simulink model "otonom_sim_lane_changing"  (R2021b)
settings: Solver=VariableStepAuto  StartTime=0.0  StopTime=100  RelTol=1e-3
libraries: simulink x16, sim3dcameralib x8, eeGeneralControl x4, robotmobilelib x2, sim3dautolib x2, slpidlib x1, sim3dlib x1
settings Model: Creator=Asus  LastModifiedBy=cx

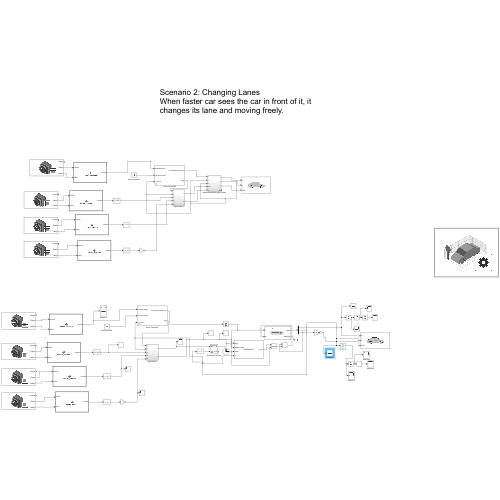
[thumbnail: Simulink's stored preview of the top-level diagram]
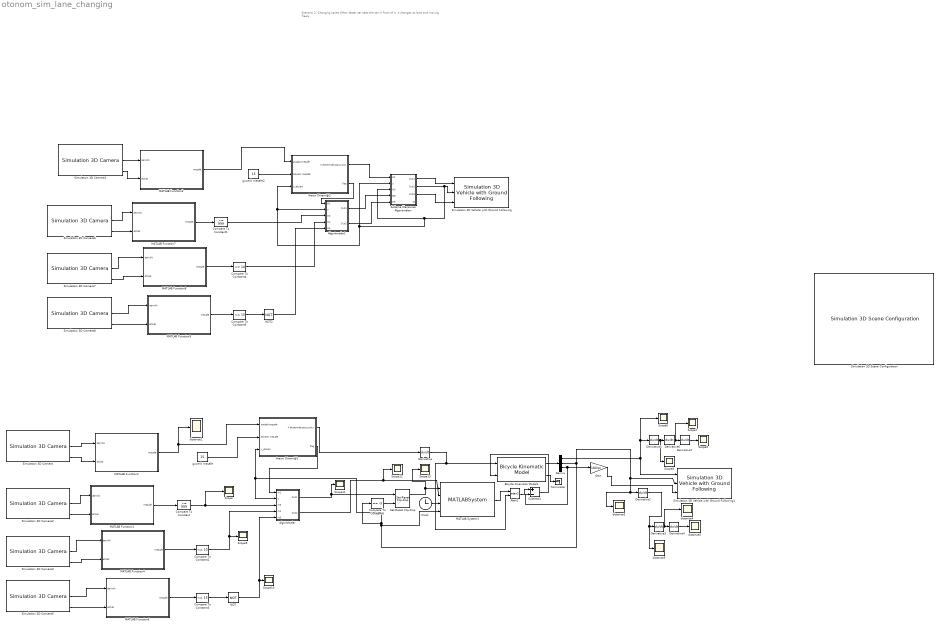
== system otonom_sim_lane_changing ==
  note: Scenario 2: Changing Lanes
      | When faster car sees the car in front of it, it changes its lane and moving freely.
  Algoritmalar : Subsystem
  Algoritmalar1 : Subsystem
  Aracın Dinamiği1 : Subsystem  mask{Konum=0, Hiz=25}
      mask prompts: Konum "Başlangıç Konumu"; Hiz "Başlangıç Hızı"
      mask TypeOptions Konum: başlangıç konumu/Value
      mask TypeOptions Hiz: başlangıç hızı/Value
  Aracın Dinamiği2 : Subsystem  mask{Konum=70, Hiz=0}
      mask prompts: Konum "Başlangıç Konumu"; Hiz "Başlangıç Hızı"
      mask TypeOptions Konum: başlangıç konumu/Value
      mask TypeOptions Hiz: başlangıç hızı/Value
  Atan2 : Trigonometry  Operator=atan2
  Bicycle Kinematic Model1 : robotmobilelib/Bicycle Kinematic Model  VehicleInputs=Vehicle Speed & Steering Angle  WheelBase=5  VehicleSpeedRange=[-inf inf]  MaxSteeringAngle=pi/4  InitialState=[0; -3; 0]  SimulateUsing=Interpreted execution
      settings: SourceProductBaseCode=RO
  Clock : Clock
  Compare To Constant : simulink/Logic and Bit Operations/Compare To Constant  relop=>=  const=999  OutDataTypeStr=boolean
  Compare To Constant1 : simulink/Logic and Bit Operations/Compare To Constant  relop=>=  const=999  OutDataTypeStr=boolean
  Compare To Constant2 : simulink/Logic and Bit Operations/Compare To Constant  relop=<=  const=10  OutDataTypeStr=boolean
  Compare To Constant3 : simulink/Logic and Bit Operations/Compare To Constant  relop=<=  const=15  OutDataTypeStr=boolean
  Compare To Constant4 : simulink/Logic and Bit Operations/Compare To Constant  relop=<=  const=10  OutDataTypeStr=boolean
  Compare To Constant5 : simulink/Logic and Bit Operations/Compare To Constant  relop=<=  const=15  OutDataTypeStr=boolean
  Compare To Constant6 : simulink/Logic and Bit Operations/Compare To Constant  relop===  const=-3  OutDataTypeStr=boolean
  Demux : Demux  Outputs=3
  Derivative{,2..7} (7 alike) : Derivative
  Gain : Gain  Gain=180/pi
  MATLAB Function1 : MATLAB Function  TreatAsAtomicUnit=on
  MATLAB Function2 : MATLAB Function  TreatAsAtomicUnit=on
  MATLAB Function3 : MATLAB Function  TreatAsAtomicUnit=on
  MATLAB Function4 : MATLAB Function  TreatAsAtomicUnit=on
  MATLAB Function6 : MATLAB Function  TreatAsAtomicUnit=on
  MATLAB Function7 : MATLAB Function  TreatAsAtomicUnit=on
  MATLAB Function8 : MATLAB Function  TreatAsAtomicUnit=on
  MATLAB Function9 : MATLAB Function  TreatAsAtomicUnit=on
  MATLAB System1 : MATLABSystem  System=SeritDegisimi  SimulateUsing=Interpreted execution
      mask Type: SeritDegisimi
      mask Display:
      | disp('SeritDegisimi');
      | port_label('input',1,'flag');
      | port_label('input',2,'sollama_flag');
      | port_label('input',3,'clock');
      | port_label('input',4,'y');
      | port_label('output',1,'y_Hiz');
  NOT : Logic  Operator=NOT  IconShape=distinctive  AllPortsSameDT=off  OutDataTypeStr=boolean
  NOT2 : Logic  Operator=NOT  IconShape=distinctive  AllPortsSameDT=off  OutDataTypeStr=boolean
  Scope{,5..13} (10 alike) : Scope
  Set-Reset Flip-Flop : eeGeneralControl/Set-Reset Flip-Flop  LabelModeActiveChoice=Discrete  UndefState=Set  Q0=0  Ts=-1
      settings: SourceProductBaseCode=PS
  Simulation 3D Camera : sim3dcameralib/Simulation 3D Camera  Priority=1  sensorTag=Sim3dSensor1  sensorId=1  sensorName=Sim3dSensor1  vehTagList={'Scene Origin';'SimulinkVehicle1';'SimulinkVehicle2';'SimulinkVehicle3'}  vehTag=SimulinkVehicle2  mountLoc=Front bumper  offsetFlag=off  tmountOffset=[4.848, 0.786, 0]  extTmount=off  rmountOffset=[0, 0, 0]  extRmount=off  FocalLength=[1109, 1109]  OpticalCenter=[640, 360]  ImageSize=[720, 1280]  RadialDistortion=[0, 0]  TangentialDistortion=[0, 0]  SensorSkew=0  DepthOutportEnabled=on  SemanticOutportEnabled=on  TransformOutportEnabled=off  SampleTime=0.1  mountPoint=[2.42400002479553 0 0.5]  mountOrientation=[0 0 0]  aMode=3  ID=1
      settings: SourceProductBaseCode=AE,DR,UV,VE
  Simulation 3D Camera1 : sim3dcameralib/Simulation 3D Camera  Priority=1  sensorTag=Sim3dSensor2  sensorId=2  sensorName=Sim3dSensor2  vehTagList={'Scene Origin';'SimulinkVehicle1';'SimulinkVehicle2'}  vehTag=SimulinkVehicle1  mountLoc=Front bumper  offsetFlag=off  tmountOffset=[0, 0, 1.2]  extTmount=off  rmountOffset=[0, 0, 0]  extRmount=off  FocalLength=[1109, 1109]  OpticalCenter=[640, 360]  ImageSize=[720, 1280]  RadialDistortion=[0, 0]  TangentialDistortion=[0, 0]  SensorSkew=0  DepthOutportEnabled=on  SemanticOutportEnabled=on  TransformOutportEnabled=off  SampleTime=0.1  mountPoint=[2.42400002479553 0 0.5]  mountOrientation=[0 0 0]  aMode=3  ID=2
      settings: SourceProductBaseCode=AE,DR,UV,VE
  Simulation 3D Camera2 : sim3dcameralib/Simulation 3D Camera  Priority=1  sensorTag=Sim3dSensor3  sensorId=3  sensorName=Sim3dSensor3  vehTagList={'Scene Origin';'SimulinkVehicle1';'SimulinkVehicle2'}  vehTag=SimulinkVehicle2  mountLoc=Right mirror  offsetFlag=on  tmountOffset=[-2, 0, 0]  extTmount=off  rmountOffset=[0, -90, -90]  extRmount=off  FocalLength=[1109, 1109]  OpticalCenter=[640, 360]  ImageSize=[720, 1280]  RadialDistortion=[0, 0]  TangentialDistortion=[0, 0]  SensorSkew=0  DepthOutportEnabled=on  SemanticOutportEnabled=on  TransformOutportEnabled=off  SampleTime=0.1  mountPoint=[-1.40600001811981 0.939999997615814 1.08000004291534]  mountOrientation=[0 0 90]  aMode=3  ID=3
      settings: SourceProductBaseCode=AE,DR,UV,VE
  Simulation 3D Camera3 : sim3dcameralib/Simulation 3D Camera  Priority=1  sensorTag=Sim3dSensor4  sensorId=4  sensorName=Sim3dSensor4  vehTagList={'Scene Origin';'SimulinkVehicle1';'SimulinkVehicle2'}  vehTag=SimulinkVehicle2  mountLoc=Left mirror  offsetFlag=on  tmountOffset=[-2, 0, 0]  extTmount=off  rmountOffset=[0, -90, 90]  extRmount=off  FocalLength=[1109, 1109]  OpticalCenter=[640, 360]  ImageSize=[720, 1280]  RadialDistortion=[0, 0]  TangentialDistortion=[0, 0]  SensorSkew=0  DepthOutportEnabled=on  SemanticOutportEnabled=on  TransformOutportEnabled=off  SampleTime=0.1  mountPoint=[-1.40600001811981 -0.939999997615814 1.08000004291534]  mountOrientation=[0 0 -90]  aMode=3  ID=4
      settings: SourceProductBaseCode=AE,DR,UV,VE
  Simulation 3D Camera5 : sim3dcameralib/Simulation 3D Camera  Priority=1  sensorTag=Sim3dSensor6  sensorId=6  sensorName=Sim3dSensor6  vehTagList={'Scene Origin';'SimulinkVehicle1';'SimulinkVehicle2'}  vehTag=SimulinkVehicle2  mountLoc=Left mirror  offsetFlag=on  tmountOffset=[-2, 0, 0]  extTmount=off  rmountOffset=[0, -90, 35]  extRmount=off  FocalLength=[1109, 1109]  OpticalCenter=[640, 360]  ImageSize=[720, 1280]  RadialDistortion=[0, 0]  TangentialDistortion=[0, 0]  SensorSkew=0  DepthOutportEnabled=on  SemanticOutportEnabled=on  TransformOutportEnabled=off  SampleTime=0.1  mountPoint=[-1.40600001811981 -0.939999997615814 1.08000004291534]  mountOrientation=[0 0 -35]  aMode=3  ID=6
      settings: SourceProductBaseCode=AE,DR,UV,VE
  Simulation 3D Camera6 : sim3dcameralib/Simulation 3D Camera  Priority=1  sensorTag=Sim3dSensor7  sensorId=7  sensorName=Sim3dSensor7  vehTagList={'Scene Origin';'SimulinkVehicle1';'SimulinkVehicle2';'SimulinkVehicle3'}  vehTag=SimulinkVehicle1  mountLoc=Right mirror  offsetFlag=on  tmountOffset=[-2, 0, 0]  extTmount=off  rmountOffset=[0, -90, -90]  extRmount=off  FocalLength=[1109, 1109]  OpticalCenter=[640, 360]  ImageSize=[720, 1280]  RadialDistortion=[0, 0]  TangentialDistortion=[0, 0]  SensorSkew=0  DepthOutportEnabled=on  SemanticOutportEnabled=on  TransformOutportEnabled=off  SampleTime=0.1  mountPoint=[-1.40600001811981 0.939999997615814 1.08000004291534]  mountOrientation=[0 0 90]  aMode=3  ID=7
      settings: SourceProductBaseCode=AE,DR,UV,VE
  Simulation 3D Camera7 : sim3dcameralib/Simulation 3D Camera  Priority=1  sensorTag=Sim3dSensor8  sensorId=8  sensorName=Sim3dSensor8  vehTagList={'Scene Origin';'SimulinkVehicle1';'SimulinkVehicle2';'SimulinkVehicle3'}  vehTag=SimulinkVehicle1  mountLoc=Left mirror  offsetFlag=on  tmountOffset=[-2, 0, 0]  extTmount=off  rmountOffset=[0, -90, 90]  extRmount=off  FocalLength=[1109, 1109]  OpticalCenter=[640, 360]  ImageSize=[720, 1280]  RadialDistortion=[0, 0]  TangentialDistortion=[0, 0]  SensorSkew=0  DepthOutportEnabled=on  SemanticOutportEnabled=on  TransformOutportEnabled=off  SampleTime=0.1  mountPoint=[-1.40600001811981 -0.939999997615814 1.08000004291534]  mountOrientation=[0 0 -90]  aMode=3  ID=8
      settings: SourceProductBaseCode=AE,DR,UV,VE
  Simulation 3D Camera8 : sim3dcameralib/Simulation 3D Camera  Priority=1  sensorTag=Sim3dSensor9  sensorId=9  sensorName=Sim3dSensor9  vehTagList={'Scene Origin';'SimulinkVehicle1';'SimulinkVehicle2';'SimulinkVehicle3'}  vehTag=SimulinkVehicle1  mountLoc=Left mirror  offsetFlag=on  tmountOffset=[-2, 0, 0]  extTmount=off  rmountOffset=[0, -90, 33]  extRmount=off  FocalLength=[1109, 1109]  OpticalCenter=[640, 360]  ImageSize=[720, 1280]  RadialDistortion=[0, 0]  TangentialDistortion=[0, 0]  SensorSkew=0  DepthOutportEnabled=on  SemanticOutportEnabled=on  TransformOutportEnabled=off  SampleTime=0.1  mountPoint=[-1.40600001811981 -0.939999997615814 1.08000004291534]  mountOrientation=[0 0 -33]  aMode=3  ID=9
      settings: SourceProductBaseCode=AE,DR,UV,VE
  Simulation 3D Scene Configuration : sim3dlib/Simulation 3D Scene Configuration  Priority=0  ProjectFormat_internal=Default Scenes  ProjectFormat=Default Scenes  SceneDesc=Straight road  ProjectName=F:\MATLAB\R2021b\toolbox\shared\sim3d_projects\automotive_project\UE4\WindowsNoEditor\VehicleSimulation.exe  ScenePath=/Game/Maps/HwStrght  vehTagList={'Scene Origin';'SimulinkVehicle1';'SimulinkVehicle2';'SimulinkVehicle3'}  vehTag=SimulinkVehicle2  OpVisEn=off  Ts=0.1  EnableWindow=on  EnableWeather=off  SunAltitude=40.0  SunAzimuth=90  clouds=10  wind=1  fog=0  rain=0  sensorTag=MainCamera1  sensorId=1  sensorName=MainCamera1  mountLoc=Origin  offsetFlag=off  tmountOffset=[0, 0, 0]  rmountOffset=[0, 0, 0]  HorizontalResolution=1280  VerticalResolution=720  HorizontalFOV=60  mountPoint=[0 0 0]  mountOrientation=[0 0 0]  aMode=3  ID=1
      settings: SourceProductBaseCode=AE,DR,UV,VE
  Simulation 3D Vehicle with Ground Following : sim3dautolib/Simulation 3D Vehicle with Ground Following  Priority=-1  PassVehMesh=Sedan  PassVehMesh_Internal=Sedan  MeshPath=/MathWorksSimulation/Vehicles/Muscle/Meshes/SK_MuscleCar.SK_MuscleCar  TrackWidth=1.9  WheelBase=3  WheelRadius=0.35  VehColor=Blue  VehColor_Internal=Blue  InitialPos=[70 -3 0]  InitialRot=[0, 0, 0]  ActorName=SimulinkVehicle1  SampleTime=0.1  ActorType=SimulinkVehicle  ID=1  aMode=3  ActorTag=SimulinkVehicle1  CoordinateScheme=ISO  VehLightsControl=off  HeadlightColor=[ 1, 1, 1 ]  HighBeamIntensity=100000  LowBeamIntensity=60000  HighBeamConeAngle=70  LowBeamConeAngle=70  LeftHeadlightOrientation=[ 0, 0 ]  RightHeadlightOrientation=[ 0, 0 ]  BrakelightIntensity=500  ReverselightIntensity=500  SignallightIntensity=500  SignallightPeriod=1  SignalPulseWidth=50  TransformOutportEnabled=off
      settings: SourceProductBaseCode=AE,DR,UV,VE
  Simulation 3D Vehicle with Ground Following1 : sim3dautolib/Simulation 3D Vehicle with Ground Following  Priority=-1  PassVehMesh=Sedan  PassVehMesh_Internal=Sedan  MeshPath=/MathWorksSimulation/Vehicles/Muscle/Meshes/SK_MuscleCar.SK_MuscleCar  TrackWidth=1.9  WheelBase=3  WheelRadius=0.35  VehColor=Red  VehColor_Internal=Red  InitialPos=[0 -3 0]  InitialRot=[0, 0, 0]  ActorName=SimulinkVehicle2  SampleTime=0.1  ActorType=SimulinkVehicle  ID=2  aMode=3  ActorTag=SimulinkVehicle2  CoordinateScheme=ISO  VehLightsControl=off  HeadlightColor=[ 1, 1, 1 ]  HighBeamIntensity=100000  LowBeamIntensity=60000  HighBeamConeAngle=70  LowBeamConeAngle=70  LeftHeadlightOrientation=[ 0, 0 ]  RightHeadlightOrientation=[ 0, 0 ]  BrakelightIntensity=500  ReverselightIntensity=500  SignallightIntensity=500  SignallightPeriod=1  SignalPulseWidth=50  TransformOutportEnabled=off
      settings: SourceProductBaseCode=AE,DR,UV,VE
  Sollama Manevrası Algoritmaları : Subsystem
  Subtract1 : Sum  Inputs=+-
  Terminator : Terminator
  distance{1..5} (5 alike) : Scope
  guvenlı mesafe : Constant  Value=15
  guvenlı mesafe2 : Constant  Value=15
  wires:
  Simulation 3D Camera1/2 -> MATLAB Function3/1(derinlik)
  Simulation 3D Camera/2 -> MATLAB Function2/1(derinlik)
  MATLAB Function3/1(mesafe) -> Aracın Dinamiği2/1(aradakimesafe)
  Simulation 3D Camera1/3 -> MATLAB Function3/2(etiket)
  guvenlı mesafe/1 -> Aracın Dinamiği1/2(Güvenli mesafe)
  Aracın Dinamiği1/1(X ekseninde posizyonu) -> Derivative/1
  Clock/1 -> MATLAB System1/3
  Derivative/1 -> Bicycle Kinematic Model1/1, Atan2/2
  Bicycle Kinematic Model1/2 -> Terminator/1
  Bicycle Kinematic Model1/1 -> Demux/1
  Demux/3 -> Subtract1/2, Gain/1
  Gain/1 -> Simulation 3D Vehicle with Ground Following1/3
  Atan2/1 -> Subtract1/1
  Subtract1/1 -> Bicycle Kinematic Model1/2
  MATLAB System1/1 -> Atan2/1
  Simulation 3D Camera/3 -> MATLAB Function2/2(etiket)
  MATLAB Function2/1(mesafe) -> distance1/1, Aracın Dinamiği1/1(aradakimesafe)
  guvenlı mesafe2/1 -> Aracın Dinamiği2/2(Güvenli mesafe)
  Derivative3/1 -> distance4/1, Derivative4/1
  Derivative2/1 -> distance3/1, Derivative3/1
  Derivative4/1 -> distance5/1
  Demux/1 -> Scope6/1, Derivative5/1, Simulation 3D Vehicle with Ground Following1/1
  Derivative6/1 -> Scope7/1, Derivative7/1
  Derivative7/1 -> Scope5/1
  Derivative5/1 -> Scope8/1, Derivative6/1
  Simulation 3D Camera2/2 -> MATLAB Function1/1(derinlik)
  Simulation 3D Camera2/3 -> MATLAB Function1/2(etiket)
  MATLAB Function1/1(mesafe) -> Compare To Constant/1
  Simulation 3D Camera3/3 -> MATLAB Function4/2(etiket)
  Simulation 3D Camera3/2 -> MATLAB Function4/1(derinlik)
  MATLAB Function4/1(mesafe) -> Compare To Constant2/1
  Simulation 3D Camera5/3 -> MATLAB Function6/2(etiket)
  Simulation 3D Camera5/2 -> MATLAB Function6/1(derinlik)
  MATLAB Function6/1(mesafe) -> Compare To Constant3/1
  Demux/2 -> Compare To Constant6/1, Aracın Dinamiği1/3(y_ekseni), Algoritmalar/2(u), MATLAB System1/4, distance2/1, Derivative2/1, Simulation 3D Vehicle with Ground Following1/2
  Compare To Constant/1 -> Scope/1, Algoritmalar/3(In3)
  Algoritmalar/1(Out1) -> Scope11/1, Set-Reset Flip-Flop/1
  Aracın Dinamiği1/2(flag) -> Algoritmalar/1(In1)
  Compare To Constant2/1 -> Scope9/1, Algoritmalar/4(In4)
  Compare To Constant3/1 -> NOT/1
  Algoritmalar/2(Out2) -> MATLAB System1/2, Scope12/1
  NOT2/1 -> Algoritmalar1/5(In5)
  Compare To Constant4/1 -> Algoritmalar1/4(In4)
  Aracın Dinamiği2/2(flag) -> Algoritmalar1/1(In1)
  Compare To Constant1/1 -> Algoritmalar1/3(In3)
  Simulation 3D Camera8/3 -> MATLAB Function9/2(etiket)
  Simulation 3D Camera7/2 -> MATLAB Function8/1(derinlik)
  MATLAB Function9/1(mesafe) -> Compare To Constant5/1
  Compare To Constant5/1 -> NOT2/1
  Simulation 3D Camera6/3 -> MATLAB Function7/2(etiket)
  MATLAB Function7/1(mesafe) -> Compare To Constant1/1
  Simulation 3D Camera8/2 -> MATLAB Function9/1(derinlik)
  Simulation 3D Camera6/2 -> MATLAB Function7/1(derinlik)
  Simulation 3D Camera7/3 -> MATLAB Function8/2(etiket)
  MATLAB Function8/1(mesafe) -> Compare To Constant4/1
  NOT/1 -> Scope10/1, Algoritmalar/5(In5)
  Set-Reset Flip-Flop/1 -> Scope13/1, MATLAB System1/1
  Compare To Constant6/1 -> Set-Reset Flip-Flop/2
  Sollama Manevrası Algoritmaları/2(Out2) -> Simulation 3D Vehicle with Ground Following/2, Sollama Manevrası Algoritmaları/2(u), Algoritmalar1/2(u), Aracın Dinamiği2/3(y_ekseni), Sollama Manevrası Algoritmaları/3(In3)
  Aracın Dinamiği2/1(X ekseninde posizyonu) -> Sollama Manevrası Algoritmaları/1(In1)
  Algoritmalar1/1(Out1) -> Sollama Manevrası Algoritmaları/4(Set)
  Algoritmalar1/2(Out2) -> Sollama Manevrası Algoritmaları/5(In5)
  Sollama Manevrası Algoritmaları/1(Out1) -> Simulation 3D Vehicle with Ground Following/1
  Sollama Manevrası Algoritmaları/3(Out3) -> Simulation 3D Vehicle with Ground Following/3

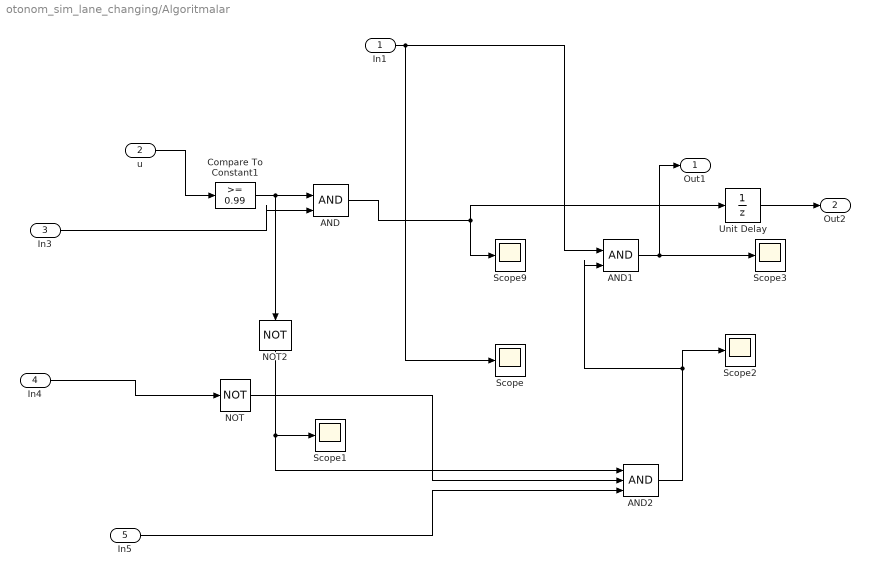
== system otonom_sim_lane_changing/Algoritmalar ==
  In1 : Inport
  u : Inport  Port=2
  In3 : Inport  Port=3
  In4 : Inport  Port=4
  In5 : Inport  Port=5
  AND : Logic  IconShape=distinctive  AllPortsSameDT=off  OutDataTypeStr=boolean
  AND1 : Logic  IconShape=distinctive  AllPortsSameDT=off  OutDataTypeStr=boolean
  AND2 : Logic  Inputs=3  IconShape=distinctive  AllPortsSameDT=off  OutDataTypeStr=boolean
  Compare To Constant1 : simulink/Logic and Bit Operations/Compare To Constant  relop=>=  const=0.99  OutDataTypeStr=boolean
  NOT : Logic  Operator=NOT  IconShape=distinctive  AllPortsSameDT=off  OutDataTypeStr=boolean
  NOT2 : Logic  Operator=NOT  IconShape=distinctive  AllPortsSameDT=off  OutDataTypeStr=boolean
  Scope{,1..3,9} (5 alike) : Scope
  Unit Delay : UnitDelay  SampleTime=-1  HasFrameUpgradeWarning=on
  Out1 : Outport
  Out2 : Outport  Port=2
  wires:
  AND2/1 -> Scope2/1, AND1/2
  In5/1 -> AND2/3
  NOT/1 -> AND2/2
  AND/1 -> Unit Delay/1, Scope9/1
  Compare To Constant1/1 -> AND/1, NOT2/1
  AND1/1 -> Out1/1, Scope3/1
  In1/1 -> Scope/1, AND1/1
  In3/1 -> AND/2
  NOT2/1 -> AND2/1, Scope1/1
  u/1 -> Compare To Constant1/1
  In4/1 -> NOT/1
  Unit Delay/1 -> Out2/1

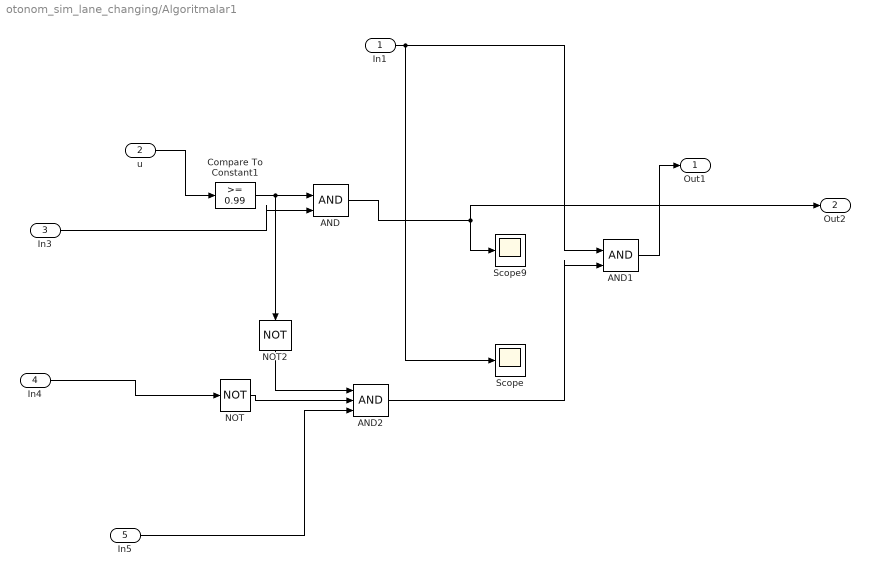
== system otonom_sim_lane_changing/Algoritmalar1 ==
  In1 : Inport
  u : Inport  Port=2
  In3 : Inport  Port=3
  In4 : Inport  Port=4
  In5 : Inport  Port=5
  AND : Logic  IconShape=distinctive  AllPortsSameDT=off  OutDataTypeStr=boolean
  AND1 : Logic  IconShape=distinctive  AllPortsSameDT=off  OutDataTypeStr=boolean
  AND2 : Logic  Inputs=3  IconShape=distinctive  AllPortsSameDT=off  OutDataTypeStr=boolean
  Compare To Constant1 : simulink/Logic and Bit Operations/Compare To Constant  relop=>=  const=0.99  OutDataTypeStr=boolean
  NOT : Logic  Operator=NOT  IconShape=distinctive  AllPortsSameDT=off  OutDataTypeStr=boolean
  NOT2 : Logic  Operator=NOT  IconShape=distinctive  AllPortsSameDT=off  OutDataTypeStr=boolean
  Scope : Scope
  Scope9 : Scope
  Out1 : Outport
  Out2 : Outport  Port=2
  wires:
  AND2/1 -> AND1/2
  In5/1 -> AND2/3
  NOT/1 -> AND2/2
  AND/1 -> Out2/1, Scope9/1
  Compare To Constant1/1 -> AND/1, NOT2/1
  AND1/1 -> Out1/1
  In1/1 -> Scope/1, AND1/1
  In3/1 -> AND/2
  NOT2/1 -> AND2/1
  u/1 -> Compare To Constant1/1
  In4/1 -> NOT/1

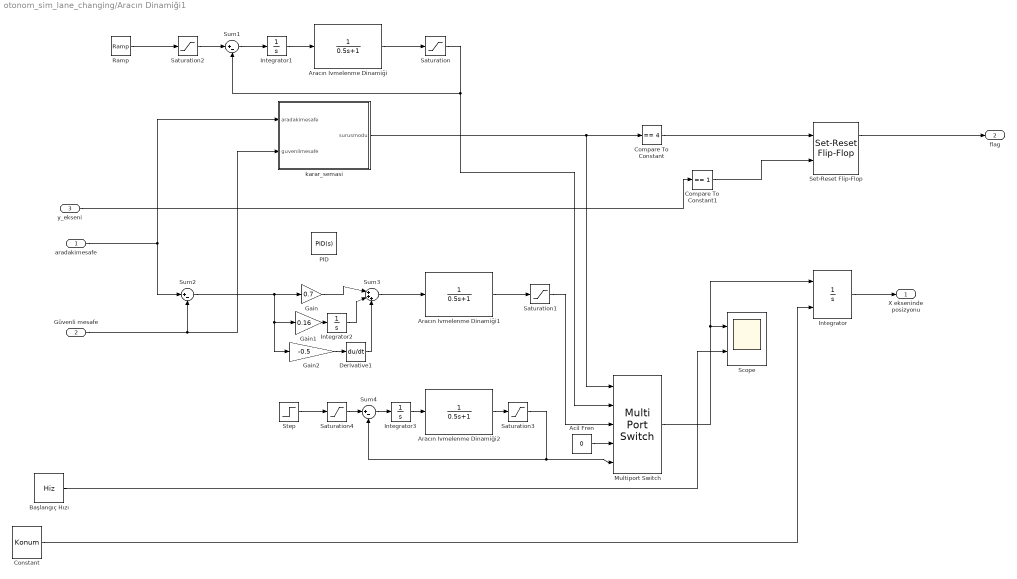
== system otonom_sim_lane_changing/Aracın Dinamiği1 ==
  aradakimesafe : Inport
  Güvenli mesafe : Inport  Port=2
  y_ekseni : Inport  Port=3
  Acil Fren : Constant  Value=0
  Aracın Ivmelenme Dinamiği : TransferFcn  Denominator=[0.5 1]
  Aracın Ivmelenme Dinamiği1 : TransferFcn  Denominator=[0.5 1]
  Aracın Ivmelenme Dinamiği2 : TransferFcn  Denominator=[0.5 1]
  Başlangıç Hızı : Constant  Value=Hiz
  Compare To Constant : simulink/Logic and Bit Operations/Compare To Constant  relop===  const=4  OutDataTypeStr=boolean
  Compare To Constant1 : simulink/Logic and Bit Operations/Compare To Constant  relop===  const=1  OutDataTypeStr=boolean
  Constant : Constant  Value=Konum
  Derivative1 : Derivative
  Gain : Gain  Gain=0.7
  Gain1 : Gain  Gain=0.16
  Gain2 : Gain  Gain=-0.5
  Integrator : Integrator  InitialConditionSource=external
  Integrator1 : Integrator
  Integrator2 : Integrator
  Integrator3 : Integrator
  Multiport Switch : MultiPortSwitch  Inputs=4
  PID : slpidlib/PID Controller  Controller=PID  Form=Parallel  TimeDomain=Continuous-time  UseExternalTs=off  SampleTime=-1  IntegratorMethod=Forward Euler  FilterMethod=Forward Euler  ControllerParametersSource=internal  P=0.955006190802503  I=0.147781151830833  D=0.621561566817517  UseFilter=on  N=108.84075962301  TunerSelectOption=Transfer Function Based (PID Tuner App)  InitialConditionSource=internal  InitialConditionForIntegrator=0  InitialConditionForFilter=0  DifferentiatorICPrevScaledInput=0  ExternalReset=none  TrackingMode=off  Kt=1  LimitOutput=off  SatLimitsSource=internal  UpperSaturationLimit=inf  LowerSaturationLimit=-inf  LinearizeAsGain=on  AntiWindupMode=none  Kb=1  POutMin=[]  POutMax=[]  IOutMin=[]  IOutMax=[]  DOutMin=[]  DOutMax=[]  NOutMin=[]  NOutMax=[]  SumOutMin=[]  SumOutMax=[]  SaturationOutMin=[]  SaturationOutMax=[]  PParamMin=[]  PParamMax=[]  IParamMin=[]  IParamMax=[]  DParamMin=[]  DParamMax=[]  NParamMin=[]  NParamMax=[]  KbParamMin=[]  KbParamMax=[]  KtParamMin=[]  KtParamMax=[]  KbOutMin=[]  KbOutMax=[]  KtOutMin=[]  KtOutMax=[]  IntegratorOutMin=[]  IntegratorOutMax=[]  FilterOutMin=[]  FilterOutMax=[]  SumI1OutMin=[]  SumI1OutMax=[]  SumI2OutMin=[]  SumI2OutMax=[]  SumI3OutMin=[]  SumI3OutMax=[]  SumI4OutMin=[]  SumI4OutMax=[]  SumDOutMin=[]  SumDOutMax=[]  DifferentiatorOutMin=[]  DifferentiatorOutMax=[]  FilterDiffOutCoefMin=[]  FilterDiffOutCoefMax=[]  ReciprocalOutMin=[]  ReciprocalOutMax=[]  SumDenOutMin=[]  SumDenOutMax=[]  SumNumOutMin=[]  SumNumOutMax=[]  DivideOutMin=[]  DivideOutMax=[]  UdiffTsProdOutMin=[]  UdiffTsProdOutMax=[]  NTsProdOutMin=[]  NTsProdOutMax=[]  UintegralTsProdOutMin=[]  UintegralTsProdOutMax=[]  UngainTsProdOutMin=[]  UngainTsProdOutMax=[]  IntegratorContinuousStateAttributes=''  IntegratorStateMustResolveToSignalObject=off  IntegratorRTWStateStorageClass=Auto  FilterContinuousStateAttributes=''  FilterStateMustResolveToSignalObject=off  FilterRTWStateStorageClass=Auto  ParallelPVariant=InternalParameters  IdealPVariant=Disabled  IVariant=InternalParameters  DVariant=InternalParameters  IntegratorVariant=Continuous  SatVariant=Disabled  AWVariant=Passthrough  PCopyVariant=Disabled  TRVariant=Disabled  FdbkBlocksVariant=Forward  IdealPFdbkVariant=Disabled  SatFdbkVariant=Disabled  DerivativeFilterVariant=ContFilter  NVariant=InternalParameters  NCopyVariant=Disabled  FilterICVariant=InternalICsFilter  IntegratorICVariant=InternalICs  ExternalResetVariant=Disabled  TRSumVariant=Passthrough  SumFdbkVariant=Disabled  SumVariant=Sum_PID  TsampFilterVariant=InternalTs  TsampNgainVariant=Passthrough  TsampIntegralVariant=Passthrough  ExternalSaturationOutDataTypeStr=Inherit: Same as second input
  Ramp : simulink/Sources/Ramp  slope=1  start=0  InitialOutput=Hiz
  Saturation : Saturate  UpperLimit=90
  Saturation1 : Saturate  UpperLimit=90
  Saturation2 : Saturate  UpperLimit=30
  Saturation3 : Saturate  UpperLimit=90
  Saturation4 : Saturate  UpperLimit=50
  Scope : Scope  NumInputPorts=2
  Set-Reset Flip-Flop : eeGeneralControl/Set-Reset Flip-Flop  LabelModeActiveChoice=Discrete  UndefState=Set  Q0=0  Ts=-1
      settings: SourceProductBaseCode=PS
  Step : Step  After=25  SampleTime=0
  Sum1 : Sum  Inputs=|+-
  Sum2 : Sum  Inputs=|+-
  Sum3 : Sum  Inputs=|+++
  Sum4 : Sum  Inputs=|+-
  karar_semasi : Stateflow chart  TreatAsAtomicUnit=on
  X ekseninde posizyonu : Outport
  flag : Outport  Port=2
  wires:
  karar_semasi/1(surusmodu) -> Compare To Constant/1, Multiport Switch/1
  Başlangıç Hızı/1 -> Scope/2
  Multiport Switch/1 -> Integrator/1, Scope/1
  Saturation/1 -> Multiport Switch/2, Sum1/2
  Acil Fren/1 -> Multiport Switch/4
  Integrator/1 -> X ekseninde posizyonu/1
  Constant/1 -> Integrator/2
  Saturation1/1 -> Multiport Switch/3
  Aracın Ivmelenme Dinamiği/1 -> Saturation/1
  Aracın Ivmelenme Dinamiği1/1 -> Saturation1/1
  Güvenli mesafe/1 -> karar_semasi/2(guvenlimesafe), Sum2/2
  aradakimesafe/1 -> karar_semasi/1(aradakimesafe), Sum2/1
  Sum1/1 -> Integrator1/1
  Integrator1/1 -> Aracın Ivmelenme Dinamiği/1
  Saturation2/1 -> Sum1/1
  Ramp/1 -> Saturation2/1
  Compare To Constant/1 -> Set-Reset Flip-Flop/1
  Set-Reset Flip-Flop/1 -> flag/1
  Derivative1/1 -> Sum3/3
  Gain1/1 -> Integrator2/1
  Integrator2/1 -> Sum3/2
  Sum2/1 -> Gain/1, Gain1/1, Gain2/1
  Gain/1 -> Sum3/1
  Gain2/1 -> Derivative1/1
  Sum3/1 -> Aracın Ivmelenme Dinamiği1/1
  Integrator3/1 -> Aracın Ivmelenme Dinamiği2/1
  Saturation4/1 -> Sum4/1
  Sum4/1 -> Integrator3/1
  Saturation3/1 -> Sum4/2, Multiport Switch/5
  Aracın Ivmelenme Dinamiği2/1 -> Saturation3/1
  Step/1 -> Saturation4/1
  y_ekseni/1 -> Compare To Constant1/1
  Compare To Constant1/1 -> Set-Reset Flip-Flop/2

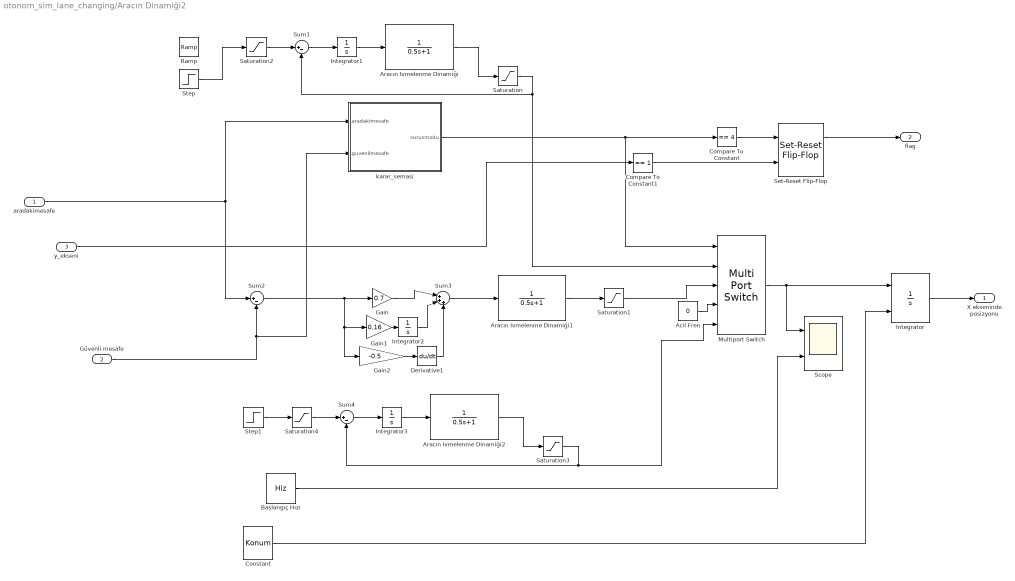
== system otonom_sim_lane_changing/Aracın Dinamiği2 ==
  aradakimesafe : Inport
  Güvenli mesafe : Inport  Port=2
  y_ekseni : Inport  Port=3
  Acil Fren : Constant  Value=0
  Aracın Ivmelenme Dinamiği : TransferFcn  Denominator=[0.5 1]
  Aracın Ivmelenme Dinamiği1 : TransferFcn  Denominator=[0.5 1]
  Aracın Ivmelenme Dinamiği2 : TransferFcn  Denominator=[0.5 1]
  Başlangıç Hızı : Constant  Value=Hiz
  Compare To Constant : simulink/Logic and Bit Operations/Compare To Constant  relop===  const=4  OutDataTypeStr=boolean
  Compare To Constant1 : simulink/Logic and Bit Operations/Compare To Constant  relop===  const=1  OutDataTypeStr=boolean
  Constant : Constant  Value=Konum
  Derivative1 : Derivative
  Gain : Gain  Gain=0.7
  Gain1 : Gain  Gain=0.16
  Gain2 : Gain  Gain=-0.5
  Integrator : Integrator  InitialConditionSource=external
  Integrator1 : Integrator
  Integrator2 : Integrator
  Integrator3 : Integrator
  Multiport Switch : MultiPortSwitch  Inputs=4
  Ramp : simulink/Sources/Ramp  slope=1  start=0  InitialOutput=Hiz
  Saturation : Saturate  UpperLimit=90
  Saturation1 : Saturate  UpperLimit=90
  Saturation2 : Saturate  UpperLimit=30
  Saturation3 : Saturate  UpperLimit=90
  Saturation4 : Saturate  UpperLimit=50
  Scope : Scope  NumInputPorts=2
  Set-Reset Flip-Flop : eeGeneralControl/Set-Reset Flip-Flop  LabelModeActiveChoice=Discrete  UndefState=Set  Q0=0  Ts=-1
      settings: SourceProductBaseCode=PS
  Step : Step  After=25  SampleTime=0
  Step1 : Step  After=25  SampleTime=0
  Sum1 : Sum  Inputs=|+-
  Sum2 : Sum  Inputs=|+-
  Sum3 : Sum  Inputs=|+++
  Sum4 : Sum  Inputs=|+-
  karar_semasi : Stateflow chart  TreatAsAtomicUnit=on
  X ekseninde posizyonu : Outport
  flag : Outport  Port=2
  wires:
  karar_semasi/1(surusmodu) -> Compare To Constant/1, Multiport Switch/1
  Başlangıç Hızı/1 -> Scope/2
  Multiport Switch/1 -> Integrator/1, Scope/1
  Saturation/1 -> Multiport Switch/2, Sum1/2
  Acil Fren/1 -> Multiport Switch/4
  Integrator/1 -> X ekseninde posizyonu/1
  Constant/1 -> Integrator/2
  Saturation1/1 -> Multiport Switch/3
  Aracın Ivmelenme Dinamiği/1 -> Saturation/1
  Aracın Ivmelenme Dinamiği1/1 -> Saturation1/1
  aradakimesafe/1 -> karar_semasi/1(aradakimesafe), Sum2/1
  Sum1/1 -> Integrator1/1
  Integrator1/1 -> Aracın Ivmelenme Dinamiği/1
  Saturation2/1 -> Sum1/1
  Step/1 -> Saturation2/1
  Güvenli mesafe/1 -> karar_semasi/2(guvenlimesafe), Sum2/2
  Compare To Constant/1 -> Set-Reset Flip-Flop/1
  Set-Reset Flip-Flop/1 -> flag/1
  Compare To Constant1/1 -> Set-Reset Flip-Flop/2
  y_ekseni/1 -> Compare To Constant1/1
  Saturation4/1 -> Sum4/1
  Aracın Ivmelenme Dinamiği2/1 -> Saturation3/1
  Step1/1 -> Saturation4/1
  Sum4/1 -> Integrator3/1
  Saturation3/1 -> Multiport Switch/5, Sum4/2
  Integrator3/1 -> Aracın Ivmelenme Dinamiği2/1
  Sum2/1 -> Gain/1, Gain1/1, Gain2/1
  Gain/1 -> Sum3/1
  Gain1/1 -> Integrator2/1
  Gain2/1 -> Derivative1/1
  Integrator2/1 -> Sum3/2
  Derivative1/1 -> Sum3/3
  Sum3/1 -> Aracın Ivmelenme Dinamiği1/1

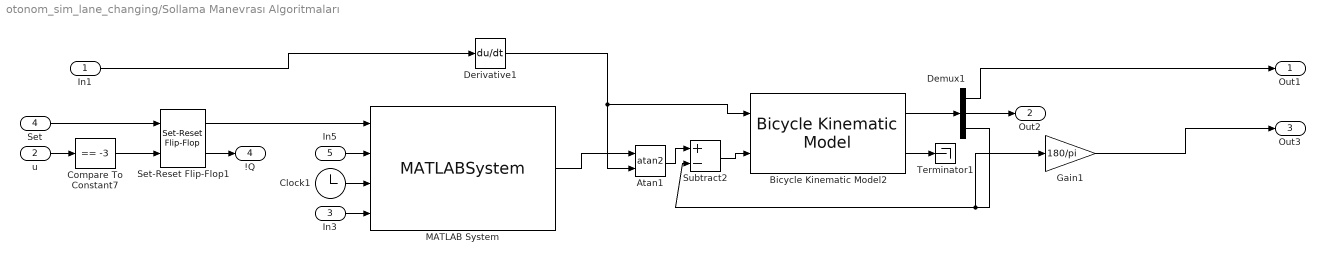
== system otonom_sim_lane_changing/Sollama Manevrası Algoritmaları ==
  In1 : Inport
  u : Inport  Port=2
  In3 : Inport  Port=3
  Set : Inport  Port=4
  In5 : Inport  Port=5
  Atan1 : Trigonometry  Operator=atan2
  Bicycle Kinematic Model2 : robotmobilelib/Bicycle Kinematic Model  VehicleInputs=Vehicle Speed & Steering Angle  WheelBase=5  VehicleSpeedRange=[-inf inf]  MaxSteeringAngle=pi/4  InitialState=[70; -3; 0]  SimulateUsing=Interpreted execution
      settings: SourceProductBaseCode=RO
  Clock1 : Clock
  Compare To Constant7 : simulink/Logic and Bit Operations/Compare To Constant  relop===  const=-3  OutDataTypeStr=boolean
  Demux1 : Demux  Outputs=3
  Derivative1 : Derivative
  Gain1 : Gain  Gain=180/pi
  MATLAB System : MATLABSystem  System=SeritDegisimi  SimulateUsing=Interpreted execution
      mask Type: SeritDegisimi
      mask Display:
      | disp('SeritDegisimi');
      | port_label('input',1,'flag');
      | port_label('input',2,'sollama_flag');
      | port_label('input',3,'clock');
      | port_label('input',4,'y');
      | port_label('output',1,'y_Hiz');
  Set-Reset Flip-Flop1 : eeGeneralControl/Set-Reset Flip-Flop  LabelModeActiveChoice=Discrete  UndefState=Set  Q0=0  Ts=-1
      settings: SourceProductBaseCode=PS
  Subtract2 : Sum  Inputs=+-
  Terminator1 : Terminator
  Out1 : Outport
  Out2 : Outport  Port=2
  Out3 : Outport  Port=3
  !Q : Outport  Port=4
  wires:
  Subtract2/1 -> Bicycle Kinematic Model2/2
  Demux1/1 -> Out1/1
  Derivative1/1 -> Bicycle Kinematic Model2/1, Atan1/2
  u/1 -> Compare To Constant7/1
  In5/1 -> MATLAB System/2
  Demux1/3 -> Subtract2/2, Gain1/1
  Demux1/2 -> Out2/1
  Atan1/1 -> Subtract2/1
  Bicycle Kinematic Model2/1 -> Demux1/1
  Bicycle Kinematic Model2/2 -> Terminator1/1
  Set-Reset Flip-Flop1/2 -> !Q/1
  MATLAB System/1 -> Atan1/1
  Gain1/1 -> Out3/1
  Clock1/1 -> MATLAB System/3
  Compare To Constant7/1 -> Set-Reset Flip-Flop1/2
  Set-Reset Flip-Flop1/1 -> MATLAB System/1
  In1/1 -> Derivative1/1
  In3/1 -> MATLAB System/4
  Set/1 -> Set-Reset Flip-Flop1/1

== matlab function otonom_sim_lane_changing/MATLAB Function6 ==
  data: derinlik input; etiket input; mesafe output
function mesafe   = mesafe_saptama( derinlik,etiket)
        
pixel_bazli_mesafe = zeros(720,1280);
pixel_bazli_mesafe(:) = 1000;

for m = 1:1:720
    for n = 1:1:1280
        if etiket(m,n) == 10
            pixel_bazli_mesafe(m,n) = derinlik(m,n);
        end
         if etiket(m,n) == 71 && derinlik(m,n) == 5
            pixel_bazli_mesafe(m,n) = 5;
        end
    end
end

mesafe = min(pixel_bazli_mesafe, [], 'all');

        
end

== matlab function otonom_sim_lane_changing/MATLAB Function7 ==
  data: derinlik input; etiket input; mesafe output
function mesafe   = mesafe_saptama( derinlik,etiket)
        
pixel_bazli_mesafe = zeros(720,1280);
pixel_bazli_mesafe(:) = 1000;

for m = 1:1:720
    for n = 1:1:1280
        if etiket(m,n) == 10
            pixel_bazli_mesafe(m,n) = derinlik(m,n);
        end
         if etiket(m,n) == 71 && derinlik(m,n) == 5
            pixel_bazli_mesafe(m,n) = 5;
        end
    end
end

mesafe = min(pixel_bazli_mesafe, [], 'all');

        
end

== matlab function otonom_sim_lane_changing/MATLAB Function8 ==
  data: derinlik input; etiket input; mesafe output
function mesafe   = mesafe_saptama( derinlik,etiket)
        
pixel_bazli_mesafe = zeros(720,1280);
pixel_bazli_mesafe(:) = 1000;

for m = 1:1:720
    for n = 1:1:1280
        if etiket(m,n) == 10
            pixel_bazli_mesafe(m,n) = derinlik(m,n);
        end
         if etiket(m,n) == 71 && derinlik(m,n) == 5
            pixel_bazli_mesafe(m,n) = 5;
        end
    end
end

mesafe = min(pixel_bazli_mesafe, [], 'all');

        
end

== matlab function otonom_sim_lane_changing/MATLAB Function9 ==
  data: derinlik input; etiket input; mesafe output
function mesafe   = mesafe_saptama( derinlik,etiket)
        
pixel_bazli_mesafe = zeros(720,1280);
pixel_bazli_mesafe(:) = 1000;

for m = 1:1:720
    for n = 1:1:1280
        if etiket(m,n) == 10
            pixel_bazli_mesafe(m,n) = derinlik(m,n);
        end
         if etiket(m,n) == 71 && derinlik(m,n) == 5
            pixel_bazli_mesafe(m,n) = 5;
        end
    end
end

mesafe = min(pixel_bazli_mesafe, [], 'all');

        
end

== stateflow chart otonom_sim_lane_changing/Aracın Dinamiği2/karar_semasi ==
  state SeritDegisimi
    entry:
    surusmodu = 4;
  state SerbestSurusModu
    entry:
    surusmodu = 1;
  state AracTakipModu
    entry:
    surusmodu = 2;
  state acilfren
    entry:
    surusmodu = 3;
  SeritDegisimi -> SerbestSurusModu : [abs(aradakimesafe-guvenlimesafe)>10]
  AracTakipModu -> SeritDegisimi [order 2] : [abs(aradakimesafe-guvenlimesafe)<=1]
  (default) -> SerbestSurusModu
  AracTakipModu -> SerbestSurusModu [order 1] : [aradakimesafe>33]
  AracTakipModu -> acilfren [order 3] : [aradakimesafe<=5]
  acilfren -> AracTakipModu : [aradakimesafe>8]
  SerbestSurusModu -> AracTakipModu [order 1] : [aradakimesafe>0 && aradakimesafe<=33]
  SerbestSurusModu -> acilfren [order 2] : [aradakimesafe <= 5 && aradakimesafe > 0]
  data: surusmodu output; aradakimesafe input; guvenlimesafe input

== stateflow chart otonom_sim_lane_changing/Aracın Dinamiği1/karar_semasi ==
  state SeritDegisimi
    entry:
    surusmodu = 4;
  state SerbestSurusModu
    entry:
    surusmodu = 1;
  state AracTakipModu
    entry:
    surusmodu = 2;
  state acilfren
    entry:
    surusmodu = 3;
  SeritDegisimi -> SerbestSurusModu : [abs(aradakimesafe-guvenlimesafe)>10]
  AracTakipModu -> SeritDegisimi [order 2] : [abs(aradakimesafe-guvenlimesafe)<=1]
  (default) -> SerbestSurusModu
  AracTakipModu -> SerbestSurusModu [order 1] : [aradakimesafe>33]
  AracTakipModu -> acilfren [order 3] : [aradakimesafe<=5]
  acilfren -> AracTakipModu : [aradakimesafe>8]
  SerbestSurusModu -> AracTakipModu [order 1] : [aradakimesafe>0 && aradakimesafe<=33]
  SerbestSurusModu -> acilfren [order 2] : [aradakimesafe <= 5 && aradakimesafe > 0]
  data: surusmodu output; aradakimesafe input; guvenlimesafe input

== matlab function otonom_sim_lane_changing/MATLAB Function2 ==
  data: derinlik input; etiket input; mesafe output
function mesafe   = mesafe_saptama( derinlik,etiket)
        
pixel_bazli_mesafe = zeros(720,1280);
pixel_bazli_mesafe(:) = 1000;

for m = 1:1:720
    for n = 620:1:660
        if etiket(m,n) == 10
            pixel_bazli_mesafe(m,n) = derinlik(m,n);
        end
         if etiket(m,n) == 71 && derinlik(m,n) == 5
            pixel_bazli_mesafe(m,n) = 5;
        end
    end
end

mesafe = min(pixel_bazli_mesafe, [], 'all');

        
end

== matlab function otonom_sim_lane_changing/MATLAB Function1 ==
  data: derinlik input; etiket input; mesafe output
function mesafe   = mesafe_saptama( derinlik,etiket)
        
pixel_bazli_mesafe = zeros(720,1280);
pixel_bazli_mesafe(:) = 1000;

for m = 1:1:720
    for n = 1:1:1280
        if etiket(m,n) == 10
            pixel_bazli_mesafe(m,n) = derinlik(m,n);
        end
         if etiket(m,n) == 71 && derinlik(m,n) == 5
            pixel_bazli_mesafe(m,n) = 5;
        end
    end
end

mesafe = min(pixel_bazli_mesafe, [], 'all');

        
end

== matlab function otonom_sim_lane_changing/MATLAB Function3 ==
  data: derinlik input; etiket input; mesafe output
function mesafe   = mesafe_saptama( derinlik,etiket)
        
pixel_bazli_mesafe = zeros(720,1280);
pixel_bazli_mesafe(:) = 1000;

for m = 1:1:720
    for n = 620:1:660
        if etiket(m,n) == 10
            pixel_bazli_mesafe(m,n) = derinlik(m,n);
        end
         if etiket(m,n) == 71 && derinlik(m,n) == 5
            pixel_bazli_mesafe(m,n) = 5;
        end
    end
end

mesafe = min(pixel_bazli_mesafe, [], 'all');

        
end

== matlab function otonom_sim_lane_changing/MATLAB Function4 ==
  data: derinlik input; etiket input; mesafe output
function mesafe   = mesafe_saptama( derinlik,etiket)
        
pixel_bazli_mesafe = zeros(720,1280);
pixel_bazli_mesafe(:) = 1000;

for m = 1:1:720
    for n = 1:1:1280
        if etiket(m,n) == 10
            pixel_bazli_mesafe(m,n) = derinlik(m,n);
        end
         if etiket(m,n) == 71 && derinlik(m,n) == 5
            pixel_bazli_mesafe(m,n) = 5;
        end
    end
end

mesafe = min(pixel_bazli_mesafe, [], 'all');

        
end
